simulink model "Modello_LQG_lineare"  (R2022b)
settings: Solver=VariableStepAuto  StartTime=0.0  StopTime=60  RelTol=1e-3
values from neighbouring files (symbols this model uses):
  A_tot = [A_nom B_nom*C_att ... (first row only)    [Inizializzazione_segway.m]    (also in LQG_controller.m = load("Matrici spazio di stato.mat","A_tot").A_tot; Matrici spazio di stato.mat = [0 79.8818966561 0 0 1 0 0 0 0 -0.384250591166 -200 0 ... (1)
  B_tot = [zeros(2,2); B_att]    [Inizializzazione_segway.m]    (also in LQG_controller.m = load("Matrici spazio di stato.mat","B_tot").B_tot; Matrici spazio di stato.mat = [0  0; 0  0; 894.427191  0; 0  894.427191])
  C_tot = [C_nom zeros(2,2)]    [Inizializzazione_segway.m]    (also in LQG_controller.m = load("Matrici spazio di stato.mat","C_tot").C_tot; Matrici spazio di stato.mat = [1  0  0  0; 0  1  0  0])
  D_tot = zeros(2,2)    [Inizializzazione_segway.m]    (also in LQG_controller.m = load("Matrici spazio di stato.mat","D_tot").D_tot; Matrici spazio di stato.mat = [0  0; 0  0])
  K = -lqr(A_tot,B_tot,Qr,Rr)    [LQG_controller.m]
  Qk = 0.01*diag([1 1])    [LQG_controller.m]
  Rk = (0.035)^2*diag([1 1])    [LQG_controller.m]
undefined symbols (not defined in the file or in its folder): Continuous, Time
libraries: simulink x4, ctrlSharedLib x1
settings Model: Creator=anton  LastModifiedBy=mircocalzaretta

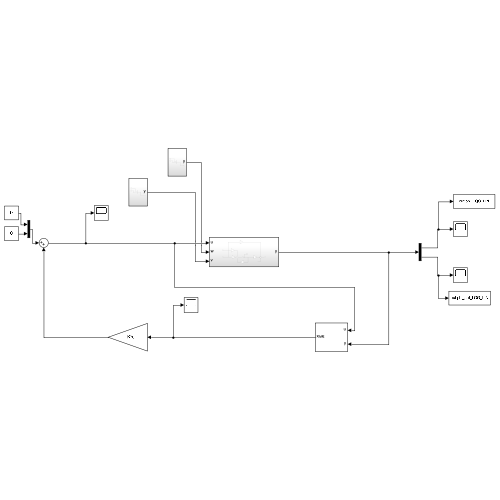
[thumbnail: Simulink's stored preview of the top-level diagram]
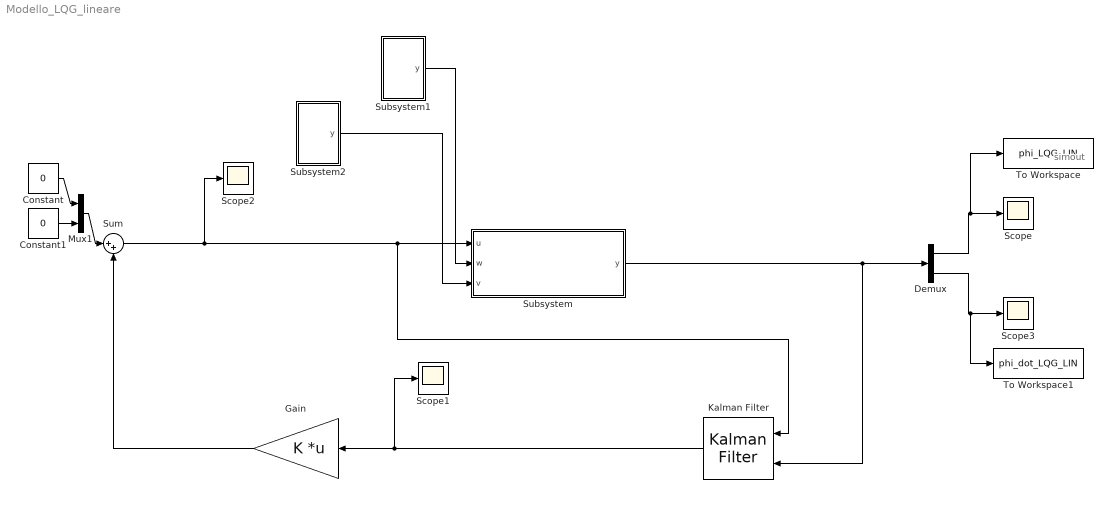
== system Modello_LQG_lineare ==
  note: simout
  Constant : Constant  Value=0
  Constant1 : Constant  Value=0
  Demux : Demux  Outputs=2
  Gain : Gain  Gain=K  Multiplication=Matrix(K*u)
  Kalman Filter : ctrlSharedLib/Kalman Filter  TimeDomain=Continuous-Time  UseCurrentEstimator=on  ModelSource=Individual A, B, C, D matrices  ModelSourceVariable=ss(0.95,1,1,0,1)  A=A_tot  B=B_tot  C=C_tot  D=D_tot  NumberOfStates=1  NumberOfInputs=1  NumberOfOutputs=1  InitialEstimateSource=Dialog  X0=[0 0 0 0]  P0=10  UseK=off  UseGH=on  NumberOfProcessNoiseInputs=1  G=B_tot  TimeInvariantG=on  H=0  TimeInvariantH=on  Q=Qk  TimeInvariantQ=on  R=Rk  TimeInvariantR=on  N=0  TimeInvariantN=on  AddInputPort=on  AddEnablePort=off  OutputEstimatedY=off  OutputP=off  Ts=-1
  Mux1 : Mux  Inputs=2
  Scope{,1..3} (4 alike) : Scope
  Subsystem : Subsystem
  Subsystem1 : Subsystem
  Subsystem2 : Subsystem
  Sum : Sum  Inputs=|++
  To Workspace : ToWorkspace  VariableName=phi_LQG_LIN  SaveFormat=Timeseries  SampleTime=-1
  To Workspace1 : ToWorkspace  VariableName=phi_dot_LQG_LIN  SaveFormat=Timeseries  SampleTime=-1
  wires:
  Sum/1 -> Scope2/1, Kalman Filter/1, Subsystem/1(u)
  Gain/1 -> Sum/2
  Subsystem/1(y) -> Demux/1, Kalman Filter/2
  Constant/1 -> Mux1/1
  Mux1/1 -> Sum/1
  Constant1/1 -> Mux1/2
  Subsystem1/1(y) -> Subsystem/2(w)
  Subsystem2/1(y) -> Subsystem/3(v)
  Kalman Filter/1 -> Scope1/1, Gain/1
  Demux/1 -> To Workspace/1, Scope/1
  Demux/2 -> To Workspace1/1, Scope3/1

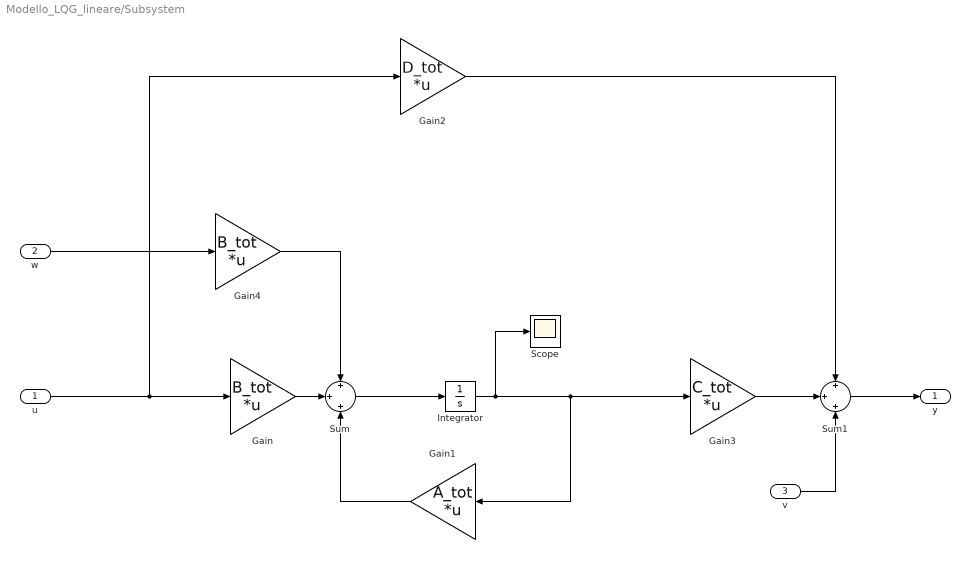
== system Modello_LQG_lineare/Subsystem ==
  u : Inport
  w : Inport  Port=2
  v : Inport  Port=3
  Gain : Gain  Gain=B_tot  Multiplication=Matrix(K*u)
  Gain1 : Gain  Gain=A_tot  Multiplication=Matrix(K*u)
  Gain2 : Gain  Gain=D_tot  Multiplication=Matrix(K*u)
  Gain3 : Gain  Gain=C_tot  Multiplication=Matrix(K*u)
  Gain4 : Gain  Gain=B_tot  Multiplication=Matrix(K*u)
  Integrator : Integrator  InitialCondition=[0 0 0 0]
  Scope : Scope
  Sum : Sum  Inputs=+|+|+
  Sum1 : Sum  Inputs=+|+|+
  y : Outport
  wires:
  Sum/1 -> Integrator/1
  Gain1/1 -> Sum/3
  u/1 -> Gain2/1, Gain/1
  Gain3/1 -> Sum1/2
  Sum1/1 -> y/1
  Gain2/1 -> Sum1/1
  Integrator/1 -> Gain3/1, Gain1/1, Scope/1
  Gain/1 -> Sum/2
  v/1 -> Sum1/3
  w/1 -> Gain4/1
  Gain4/1 -> Sum/1

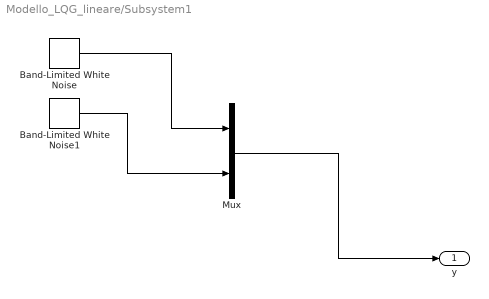
== system Modello_LQG_lineare/Subsystem1 ==
  Band-Limited White Noise : simulink/Sources/Band-Limited White Noise  Cov=[Qk(1,1)]  Ts=0.01  seed=[23341]
  Band-Limited White Noise1 : simulink/Sources/Band-Limited White Noise  Cov=[Qk(2,2)]  Ts=0.01  seed=[23341]
  Mux : Mux  Inputs=2
  y : Outport
  wires:
  Band-Limited White Noise/1 -> Mux/1
  Band-Limited White Noise1/1 -> Mux/2
  Mux/1 -> y/1

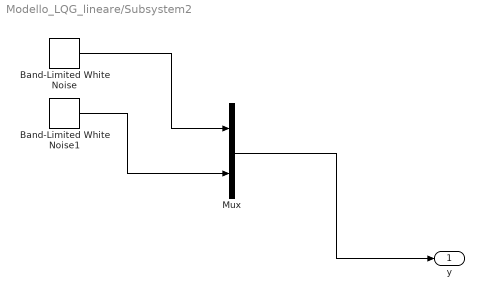
== system Modello_LQG_lineare/Subsystem2 ==
  Band-Limited White Noise : simulink/Sources/Band-Limited White Noise  Cov=[Rk(1,1)]  Ts=0.1  seed=[23341]
  Band-Limited White Noise1 : simulink/Sources/Band-Limited White Noise  Cov=[Rk(2,2)]  Ts=0.1  seed=[23341]
  Mux : Mux  Inputs=2
  y : Outport
  wires:
  Band-Limited White Noise/1 -> Mux/1
  Band-Limited White Noise1/1 -> Mux/2
  Mux/1 -> y/1
